simulink model "ball_on_beam_sim_HW_04_b"  (R2018a)
settings: Solver=ode45  StartTime=0.0  StopTime=100  MaxStep=1  RelTol=1e-3
InitFcn:
  | ball_on_beam_param
undefined symbols (not defined in the file or in its folder): ball_on_beam_animation
settings Model: Creator=canla  LastModifiedBy=canla
settings OptimizationCC: LifeSpan=inf

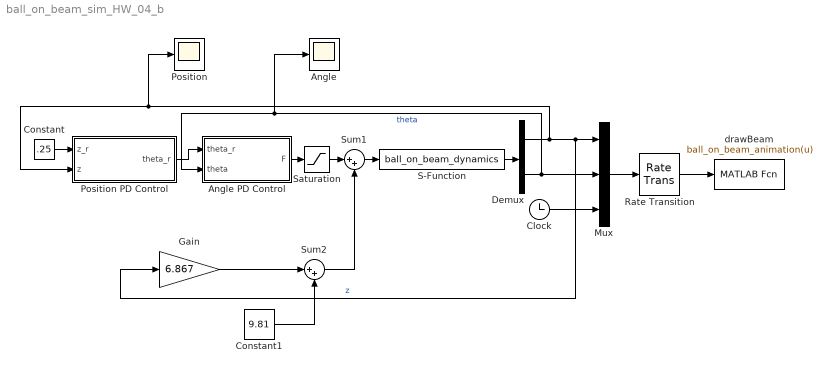
== system ball_on_beam_sim_HW_04_b ==
  Angle : Scope
  Angle PD Control : Subsystem
  Clock : Clock
  Constant : Constant  Value=.25
  Constant1 : Constant  Value=9.81
  Demux : Demux  Outputs=2
  Gain : Gain  Gain=6.867
  Mux : Mux  Inputs=3
  Position : Scope
  Position PD Control : Subsystem
  Rate Transition : RateTransition  OutPortSampleTime=Par.t_plot
  S-Function : S-Function  FunctionName=ball_on_beam_dynamics  Parameters=Par  SFunctionDeploymentMode=off  EnableBusSupport=off
  Saturation : Saturate  UpperLimit=15  LowerLimit=-15
  Sum1 : Sum  Inputs=|++
  Sum2 : Sum  Inputs=|++
  drawBeam : MATLABFcn  MATLABFcn=ball_on_beam_animation(u)  OutputDimensions=0
  wires:
  S-Function/1 -> Demux/1
  Demux/2 -> Angle/1, Angle PD Control/2(theta), Mux/2  "theta"
  Demux/1 -> Position/1, Position PD Control/2(z), Gain/1, Mux/1  "z"
  Clock/1 -> Mux/3
  Mux/1 -> Rate Transition/1
  Rate Transition/1 -> drawBeam/1
  Constant/1 -> Position PD Control/1(z_r)
  Position PD Control/1(theta_r) -> Angle PD Control/1(theta_r)
  Sum1/1 -> S-Function/1
  Gain/1 -> Sum2/1
  Constant1/1 -> Sum2/2
  Sum2/1 -> Sum1/2
  Angle PD Control/1(F) -> Saturation/1
  Saturation/1 -> Sum1/1

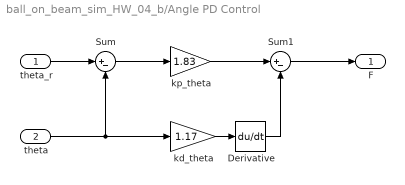
== system ball_on_beam_sim_HW_04_b/Angle PD Control ==
  theta_r : Inport
  theta : Inport  Port=2
  Derivative : Derivative
  Sum : Sum  Inputs=|+-
  Sum1 : Sum  Inputs=|+-
  kd_theta : Gain  Gain=1.17
  kp_theta : Gain  Gain=1.83
  F : Outport
  wires:
  theta_r/1 -> Sum/1
  theta/1 -> kd_theta/1, Sum/2
  Sum/1 -> kp_theta/1
  Sum1/1 -> F/1
  kp_theta/1 -> Sum1/1
  kd_theta/1 -> Derivative/1
  Derivative/1 -> Sum1/2

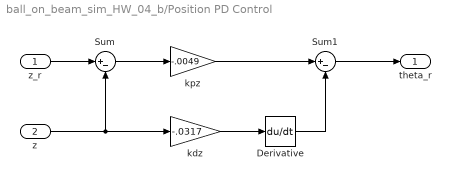
== system ball_on_beam_sim_HW_04_b/Position PD Control ==
  z_r : Inport
  z : Inport  Port=2
  Derivative : Derivative
  Sum : Sum  Inputs=|+-
  Sum1 : Sum  Inputs=|+-
  kdz : Gain  Gain=-.0317
  kpz : Gain  Gain=-.0049
  theta_r : Outport
  wires:
  z_r/1 -> Sum/1
  Sum/1 -> kpz/1
  z/1 -> Sum/2, kdz/1
  kdz/1 -> Derivative/1
  kpz/1 -> Sum1/1
  Derivative/1 -> Sum1/2
  Sum1/1 -> theta_r/1
